simulink model "SSH"  (R2020a)
settings: Solver=VariableStepAuto  StartTime=0.0  StopTime=10000  RelTol=1e-3
values from neighbouring files (symbols this model uses):
  A = [-3.94751 3.782493;0.053859 -0.054981]    [ssh.m]
  B = [0.165017 0; 0 0.001122]    [ssh.m]
  C = [1,0;0,1]    [ssh.m]
  D = [0,0;0,0]    [ssh.m]
  TGi = 1028    [ssh.m]
  TM = 501    [ssh.m]
  TS = 491    [ssh.m]
  TSi = 450    [ssh.m]
settings Model: Creator=estufab4  LastModifiedBy=estufab4

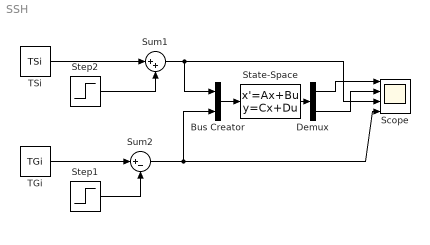
== system SSH ==
  Bus Creator : BusCreator  Inputs=2
  Demux : Demux  Outputs=2
  Scope : Scope  NumInputPorts=4
  State-Space : StateSpace  A=A  B=B  C=C  D=D  InitialCondition=[TS,TM]
  Step1 : Step  Time=6000  After=51  SampleTime=0
  Step2 : Step  Time=2000  After=22  SampleTime=0
  Sum1 : Sum  Inputs=|++
  Sum2 : Sum  Inputs=|+-
  TGi : Constant  Value=TGi
  TSi : Constant  Value=TSi
  wires:
  State-Space/1 -> Demux/1
  Bus Creator/1 -> State-Space/1
  Demux/1 -> Scope/1
  Demux/2 -> Scope/2
  TSi/1 -> Sum1/1
  Sum1/1 -> Scope/3, Bus Creator/1
  Step2/1 -> Sum1/2
  Sum2/1 -> Scope/4, Bus Creator/2
  TGi/1 -> Sum2/1
  Step1/1 -> Sum2/2
